simulink model "PIDControls"  (R2024a)
settings: Solver=VariableStepAuto  StartTime=0.0  StopTime=220  RelTol=1e-3
model workspace (MATLAB code in the model file):
  | load('DesiredPitch.mat', '-ascii');
  | load('MeasuredPitch.mat', '-ascii');
  | load('MotorPitchSpeed.mat', '-ascii');
libraries: simulink x6, slpidlib x3, mcbhdlpositiondecoderlib x3
settings Model: Creator=brend  LastModifiedBy=brend

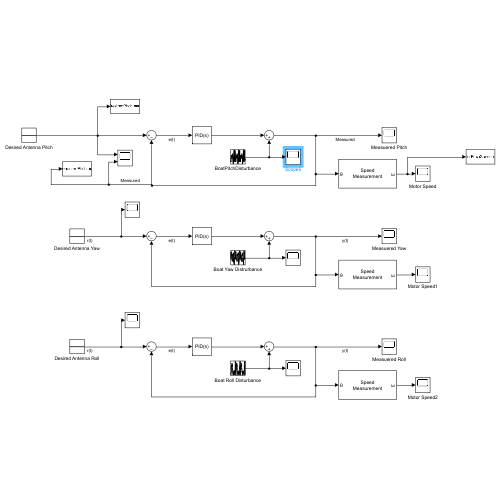
[thumbnail: Simulink's stored preview of the top-level diagram]
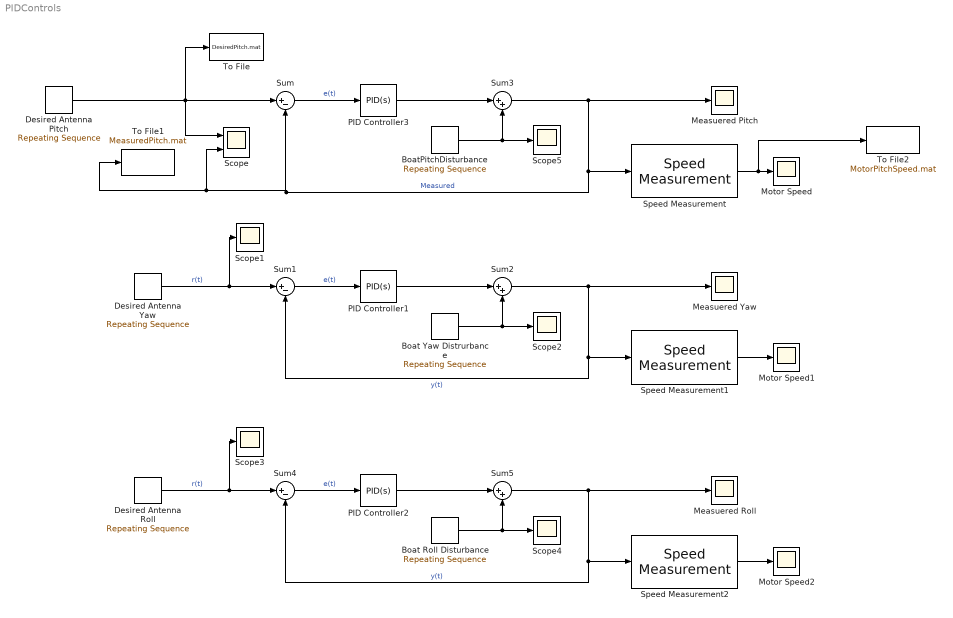
== system PIDControls ==
  Boat Roll Disturbance : simulink/Sources/Repeating Sequence  rep_seq_t=[0:219]  rep_seq_y=|
      | [-14.82
      | -14.76
      | -14.44
      | -13.69
      | -13.53
      | -13.69
      | -13.93
      | -12.12
      | -11.59
      | -10.70
      | -9.70
      | -8.71
      | -8.04
      | -7.18
      | -7.72
      | -7.28
      | -6.48
      | -6.82
      | -5.69
      | -4.25
      | -3.67
      | -2.77
      | 4.98
      | 1.24
      | 2.72
      | 3.04
      | 5.30
      | 5.55
      | 6.34
      | 5.33
      | 4.86
      | 4.27
      | 3.96
      | 3.72
      | 3.36
      | 3.85
      | 3.34
      | 3.19
      | 3.12
      | 4.38
      | 5.56
      | 6.85
      | 8.98
      | 8.41
      | 10.12
      | 10.66
      | 10.62
      | 10.05
      | 10.68
      | 10.99
      | 9.31
      | 9.86
      | 9.73
      |  9.94
      |  9.40
      |  8.03
      |  8.72
      |  8.40
      |  8.06
      |  8.71
      |  8.34
      |  8.92
      |  7.35
      | 7.33
      | 7.25
      | 6.62
      | 5.37
      | 2.19
      | 1.43
      | -3.62
      | -4.20
      | -4.94
      | -5.09
      | -4.96
      | -4.24
      | -4.35
      | -4.67
      | -4.65
      | -4.90
      | -4.35
      | -5.32
      | -6.85
      | -7.31
      | -8.65
      | -9.51
      | -9.25
      | -9.49
      | -8.63
      | -7.78
      | -7.82
      | -6.51
      | -6.54
      | -6.65
      | -6.65
      | -6.33
      | -7.93
      | -8.33
      | -10.03
      | -10.99
      | -11.75
      | -12.80
      | -12.82
      | -13.35
      | -13.70
      | -14.00
      | -14.19
      | -14.98
      | -15.90
      | -15.33
      | -15.71
      | -15.71
      | -14.54
      | -13.07
      |  -13.51
      |  -12.82
      |  -12.40
      |  -11.25
      |  -11.17
      |  -11.99
      |  -11.62
      |  -11.31
      |  -11.53
      |  -14.76
      |  -9.06
      |  -8.28
      | -7.97
      |  -7.84
      |  -8.19
      |  -8.18
      |  -9.32
      |  -10.31
      |  -11.65
      |  -12.48
      |  -13.99
      |  -13.11
      |  -14.27
      |  -13.54
      |  -14.41
      |  -13.38
      |  -9.72
      |  -7.96
      |  -6.05
      |  -5.00
      |  -5.70
      |  -5.78
      |  -5.59
      |  -5.76
      |  -5.11
      |  -5.50
      |  -5.89
      |  -5.28
      |  -5.76
      |  -5.48
      |  -5.73
      |  -6.97
      |  -6.88
      |  -7.37
      | -8.31
      | -9.30
      | -10.64
      | -11.10
      | -12.63
      | -12.95
      | -13.27
      | -13.87
      | -13.60
      | -13.99
      | -17.11
      | -13.40
      | -11.64
      | -10.60
      |  -10.77
      |  -10.26
      |  -11.02
      |  -11.54
      |  -11.51
      |  -11.68
      |  -11.79
      |  -10.58
      |  -10.79
      |  -10.15
      |  -9.59
      |  -8.36
      |  -7.25
      |  -6.32
      |  -5.45
      |  -4.09
      |  -4.25
      |  -3.73
      |  -3.28
      |  -3.67
      |  -2.62
      |  -2.80
      | -2.70
      | -2.38
      |  1.01
      |  2.23
      |  2.11
      |  4.37
      |  6.51
      |  7.00
      |  7.75
      |  8.28
      |  8.00
      |  9.87
      |  10.54
      |  10.20
      |  11.15
      |  13.65
      |  13.74
      |  14.26
      |  14.88
      |  14.77
      |  13.66
      |  12.22
      |  12.93
      |  11.12
      |  12.36
      |  12.25
      |  14.61]
  Boat Yaw Distrurbance : simulink/Sources/Repeating Sequence  rep_seq_t=[0:219]  rep_seq_y=|
      | [-5.64 
      | -4.89 
      | -3.70 
      | -2.04 
      | 0.07  
      | 2.54  
      | 5.24  
      | 7.96  
      | 10.51 
      | 12.70 
      | 14.35 
      | 15.35 
      | 15.66 
      | 15.27 
      | 14.23 
      | 12.65 
      | 10.67 
      | 8.48  
      | 6.28  
      | 4.24  
      | 2.51  
      | 1.16  
      | 0.21  
      | -0.38 
      | -0.68 
      | -0.81 
      | -0.86 
      | -0.92 
      | -1.06 
      | -1.29 
      | -1.62 
      | -1.99 
      | -2.37 
      | -2.70 
      | -2.94 
      | -3.08 
      | -3.14 
      | -3.15 
      | -3.15 
      | -3.22 
      | -3.40 
      | -3.72 
      | -4.21 
      | -4.84 
      | -5.58 
      | -6.37 
      | -7.15 
      | -7.86 
      | -8.47 
      | -8.95 
      | -9.32 
      | -9.59 
      | -9.81 
      | -10.01
      | -10.24
      | -10.51
      | -10.83
      | -11.15
      | -11.43
      | -11.58
      | -11.53
      | -11.20
      | -10.50
      | -9.40 
      | -7.90 
      | -6.02 
      | -3.83 
      | -1.47 
      | 0.92  
      | 3.18  
      | 5.15  
      | 6.72  
      | 7.81  
      | 8.39  
      | 8.48  
      | 8.16  
      | 7.53  
      | 6.73  
      | 5.90  
      | 5.18  
      | 4.67  
      | 4.44  
      | 4.50  
      | 4.81  
      |  5.31 
      |  5.88 
      |  6.43 
      | 6.86  
      | 7.10  
      | 7.14  
      | 7.01  
      | 6.76  
      | 6.49  
      | 6.29  
      | 6.25  
      | 6.43  
      | 6.85  
      |  7.45 
      |  8.17 
      |  8.87 
      |  9.43 
      |  9.75 
      |  9.75 
      |  9.40 
      |  8.75 
      |  7.89 
      |  6.98 
      |  6.21 
      |  5.73 
      |  5.71 
      |  6.20 
      |  7.21 
      |  8.61 
      |  10.22
      |  11.78
      |  13.04
      |  13.74
      |  13.69
      |  12.77
      |  10.92
      |  8.22 
      |  4.82 
      |  1.01 
      |  -2.85
      | -6.39 
      | -9.30 
      | -11.37
      | -12.50
      | -12.70
      | -12.07
      | -10.76
      | -9.00 
      | -7.06 
      | -5.22 
      | -3.72 
      | -2.76 
      | -2.46 
      | -2.85 
      | -3.92 
      | -5.58 
      | -7.68 
      | -10.06
      | -12.54
      | -14.95
      | -17.15
      | -19.00
      | -20.43
      | -21.38
      | -21.81
      | -21.71
      | -21.11
      | -20.05
      | -18.59
      | -16.85
      | -14.95
      | -13.06
      | -11.30
      | -9.79 
      | -8.61 
      | -7.77 
      | -7.20 
      | -6.82 
      | -6.46 
      | -5.97 
      | -5.21 
      | -4.05 
      | -2.43 
      | -0.34 
      |  2.13 
      |  4.88 
      |  7.73 
      |  10.50
      |  13.02
      |  15.18
      |  16.90
      |  18.15
      |  18.94
      |  19.33
      |  19.36
      |  19.09
      |  18.59
      |  17.90
      | 17.06 
      | 16.10 
      | 15.04 
      |  13.89
      |  12.67
      |  11.41
      |  10.12
      |  8.84 
      |  7.57 
      |  6.33 
      |  5.10 
      | 3.89  
      | 2.67  
      | 1.43  
      | 0.16  
      | -1.12 
      | -2.38 
      | -3.56 
      | -4.59 
      | -5.40 
      | -5.94 
      | -6.16 
      | -6.07 
      | -5.70 
      | -5.14 
      | -4.49 
      | -3.85 
      | -3.32 
      | -2.99 
      | -2.89 
      | -2.99 
      | -3.25 
      | -3.56 
      | -3.82 
      | -3.94 
      | -3.85 
      | -3.52 
      | -2.98 ]
  BoatPitchDisturbance : simulink/Sources/Repeating Sequence  rep_seq_t=[0:219]  rep_seq_y=|
      | [-6.01
      | -7.17
      | -8.05
      | -8.55
      | -8.58
      | -8.11
      | -7.17
      | -5.83
      | -4.20
      | -2.44
      | -0.69
      | 0.91 
      | 2.25 
      | 3.27 
      | 3.96 
      | 4.35 
      | 4.47 
      | 4.38 
      | 4.14 
      | 3.79 
      | 3.37 
      | 2.90 
      | 2.40 
      | 1.90 
      | 1.42 
      | 1.00 
      | 0.69 
      | 0.54 
      | 0.60 
      | 0.90 
      | 1.41 
      | 2.12 
      | 2.93 
      | 3.75 
      | 4.46 
      | 4.96 
      | 5.15 
      | 4.99 
      | 4.48 
      | 3.65 
      | 2.60 
      | 1.44 
      | 0.30 
      | -0.72
      | -1.51
      | -2.04
      | -2.28
      | -2.27
      | -2.08
      | -1.75
      | -1.37
      | -0.99
      | -0.65
      | -0.34
      | -0.07
      | 0.18 
      | 0.44 
      | 0.71 
      | 1.00 
      | 1.30 
      | 1.57 
      | 1.81 
      | 2.00 
      | 2.13 
      | 2.24 
      | 2.36 
      | 2.55 
      | 2.86 
      | 3.33 
      | 3.98 
      | 4.77 
      | 5.66 
      | 6.55 
      | 7.32 
      | 7.85 
      | 8.06 
      | 7.88 
      | 7.30 
      | 6.35 
      | 5.12 
      | 3.74 
      | 2.38 
      | 1.18 
      | 0.28 
      | -0.23
      | -0.34
      | -0.05
      | 0.53 
      | 1.29 
      | 2.08 
      | 2.77 
      | 3.23 
      | 3.36 
      | 3.12 
      | 2.49 
      | 1.50 
      | 0.20 
      | -1.33
      | -2.99
      | -4.69
      | -6.35
      | -7.88
      | -9.21
      | -10.32
      | -11.14
      | -11.75
      | -11.93
      | -11.97
      | -11.84
      | -11.45
      | -10.95
      | -10.43
      | -9.91
      | -9.38
      | -8.88
      | -8.36
      | -7.80
      | -7.13
      | -6.30
      | -5.29
      | -4.08
      | -2.73
      | -1.33
      | -0.00
      | 1.10 
      | 1.83 
      | 2.06 
      | 1.74 
      | 0.86 
      | -0.50
      | -2.18
      | -3.97
      | -5.62
      | -6.91
      | -7.63
      | -7.66
      | -6.92
      | -5.45
      | -3.34
      | -0.76
      | 2.08 
      | 4.94 
      | 7.61 
      | 9.95 
      | 11.85
      | 13.27
      | 14.22
      | 14.73
      | 14.83
      | 14.56
      | 13.93
      | 12.96
      | 11.65
      | 10.02
      | 8.09 
      | 5.93 
      | 3.63 
      | 1.33 
      | -0.81
      | -2.63
      | -4.03
      | -4.90
      | -5.23
      | -5.06
      | -4.51
      | -3.72
      | -2.89
      | -2.20
      | -1.82
      | -1.84
      | -2.32
      | -3.20
      | -4.36
      | -5.64
      | -6.84
      | -7.74
      | -8.16
      | -7.98
      | -7.12
      | -5.59
      | -3.45
      | -0.84
      | 2.04 
      | 4.96 
      | 7.69 
      | 10.02
      | 11.80
      | 12.96
      | 13.46
      | 13.33
      | 12.63
      | 11.49
      | 10.03
      | 8.41 
      | 6.80 
      | 5.31 
      | 4.05 
      | 3.07 
      | 2.35 
      | 1.86 
      | 1.50 
      | 1.18 
      | 0.81 
      | 0.32 
      | -0.31
      | -1.06
      | -1.90
      | -2.72
      | -3.42
      | -3.92
      | -4.16
      | -4.10
      | -3.80
      | -3.32
      | -2.80
      | -2.38
      | -2.20
      | -2.35
      | -2.88
      | -3.76]
  "Desired Antenna Pitch " : simulink/Sources/Repeating Sequence  rep_seq_t=[0:219]  rep_seq_y=linspace(30, 30, 220);
  Desired Antenna Roll : simulink/Sources/Repeating Sequence  rep_seq_t=[0:219]  rep_seq_y=linspace(30, 30, 220);
  Desired Antenna Yaw : simulink/Sources/Repeating Sequence  rep_seq_t=[0:219]  rep_seq_y=linspace(30, 30, 220);
  Measuered Pitch : Scope
  Measuered Roll : Scope
  Measuered Yaw : Scope
  Motor Speed : Scope
  Motor Speed1 : Scope
  Motor Speed2 : Scope
  PID Controller1 : slpidlib/PID Controller  Controller=PID  Form=Parallel  TimeDomain=Continuous-time  UseExternalTs=off  SampleTime=-1  IntegratorMethod=Forward Euler  FilterMethod=Forward Euler  ControllerParametersSource=internal  P=1  I=10  UseKiTs=off  D=0  UseExternalDerivativeSource=off  N=100  UseFilter=on  TunerSelectOption=Transfer Function Based (PID Tuner App)  InitialConditionSource=internal  InitialConditionForIntegrator=0  InitialConditionForFilter=0  DifferentiatorICPrevScaledInput=0  ExternalReset=none  TrackingMode=off  Kt=1  LimitOutput=off  SatLimitsSource=internal  UpperSaturationLimit=inf  LowerSaturationLimit=-inf  LinearizeAsGain=on  AntiWindupMode=none  Kb=1  LimitIntegrator=off  UpperIntegratorSaturationLimit=inf  LowerIntegratorSaturationLimit=-inf  POutMin=[]  POutMax=[]  IOutMin=[]  IOutMax=[]  DOutMin=[]  DOutMax=[]  NOutMin=[]  NOutMax=[]  SumOutMin=[]  SumOutMax=[]  SaturationOutMin=[]  SaturationOutMax=[]  PParamMin=[]  PParamMax=[]  IParamMin=[]  IParamMax=[]  DParamMin=[]  DParamMax=[]  NParamMin=[]  NParamMax=[]  KbParamMin=[]  KbParamMax=[]  KtParamMin=[]  KtParamMax=[]  KbOutMin=[]  KbOutMax=[]  KtOutMin=[]  KtOutMax=[]  IntegratorOutMin=[]  IntegratorOutMax=[]  FilterOutMin=[]  FilterOutMax=[]  SumI1OutMin=[]  SumI1OutMax=[]  SumI2OutMin=[]  SumI2OutMax=[]  SumI3OutMin=[]  SumI3OutMax=[]  SumI4OutMin=[]  SumI4OutMax=[]  SumDOutMin=[]  SumDOutMax=[]  DifferentiatorOutMin=[]  DifferentiatorOutMax=[]  FilterDiffOutCoefMin=[]  FilterDiffOutCoefMax=[]  ReciprocalOutMin=[]  ReciprocalOutMax=[]  SumDenOutMin=[]  SumDenOutMax=[]  SumNumOutMin=[]  SumNumOutMax=[]  DivideOutMin=[]  DivideOutMax=[]  UdiffTsProdOutMin=[]  UdiffTsProdOutMax=[]  NTsProdOutMin=[]  NTsProdOutMax=[]  UintegralTsProdOutMin=[]  UintegralTsProdOutMax=[]  UngainTsProdOutMin=[]  UngainTsProdOutMax=[]  ClampingZeroOutDataTypeStr=Inherit: Inherit via back propagation  ClampingZeroOutMin=[]  ClampingZeroOutMax=[]  FilterDenConstantOutDataTypeStr=Inherit: Inherit via back propagation  FilterDenConstantOutMin=[]  FilterDenConstantOutMax=[]  PCopyOutDataTypeStr=Inherit: Inherit via back propagation  PCopyOutMin=[]  PCopyOutMax=[]  NCopyOutDataTypeStr=Inherit: Inherit via back propagation  NCopyOutMin=[]  NCopyOutMax=[]  IntegratorContinuousStateAttributes=''  IntegratorStateMustResolveToSignalObject=off  IntegratorRTWStateStorageClass=Auto  FilterContinuousStateAttributes=''  FilterStateMustResolveToSignalObject=off  FilterRTWStateStorageClass=Auto  ParallelPVariant=InternalParameters  IdealPVariant=Disabled  IVariant=InternalParameters  DVariant=InternalParameters  IntegratorVariant=Continuous  SatVariant=Disabled  AWVariant=Passthrough  PCopyVariant=Disabled  TRVariant=Disabled  FdbkBlocksVariant=Forward  IdealPFdbkVariant=Disabled  SatFdbkVariant=Disabled  DerivativeFilterVariant=ContFilter  NVariant=InternalParameters  NCopyVariant=Disabled  FilterICVariant=InternalICsFilter  IntegratorICVariant=InternalICs  ExternalResetVariant=Disabled  TRSumVariant=Passthrough  SumFdbkVariant=Disabled  SumVariant=Sum_PID  TsampFilterVariant=InternalTs  TsampNgainVariant=Passthrough  TsampIntegralVariant=Disabled_SignalSpec  ExternalSaturationOutDataTypeStr=Inherit: Same as second input  DerivativeSourceVariant=ErrorSignal
  PID Controller2 : slpidlib/PID Controller  Controller=PID  Form=Parallel  TimeDomain=Continuous-time  UseExternalTs=off  SampleTime=-1  IntegratorMethod=Forward Euler  FilterMethod=Forward Euler  ControllerParametersSource=internal  P=1  I=10  UseKiTs=off  D=0  UseExternalDerivativeSource=off  N=100  UseFilter=on  TunerSelectOption=Transfer Function Based (PID Tuner App)  InitialConditionSource=internal  InitialConditionForIntegrator=0  InitialConditionForFilter=0  DifferentiatorICPrevScaledInput=0  ExternalReset=none  TrackingMode=off  Kt=1  LimitOutput=off  SatLimitsSource=internal  UpperSaturationLimit=inf  LowerSaturationLimit=-inf  LinearizeAsGain=on  AntiWindupMode=none  Kb=1  LimitIntegrator=off  UpperIntegratorSaturationLimit=inf  LowerIntegratorSaturationLimit=-inf  POutMin=[]  POutMax=[]  IOutMin=[]  IOutMax=[]  DOutMin=[]  DOutMax=[]  NOutMin=[]  NOutMax=[]  SumOutMin=[]  SumOutMax=[]  SaturationOutMin=[]  SaturationOutMax=[]  PParamMin=[]  PParamMax=[]  IParamMin=[]  IParamMax=[]  DParamMin=[]  DParamMax=[]  NParamMin=[]  NParamMax=[]  KbParamMin=[]  KbParamMax=[]  KtParamMin=[]  KtParamMax=[]  KbOutMin=[]  KbOutMax=[]  KtOutMin=[]  KtOutMax=[]  IntegratorOutMin=[]  IntegratorOutMax=[]  FilterOutMin=[]  FilterOutMax=[]  SumI1OutMin=[]  SumI1OutMax=[]  SumI2OutMin=[]  SumI2OutMax=[]  SumI3OutMin=[]  SumI3OutMax=[]  SumI4OutMin=[]  SumI4OutMax=[]  SumDOutMin=[]  SumDOutMax=[]  DifferentiatorOutMin=[]  DifferentiatorOutMax=[]  FilterDiffOutCoefMin=[]  FilterDiffOutCoefMax=[]  ReciprocalOutMin=[]  ReciprocalOutMax=[]  SumDenOutMin=[]  SumDenOutMax=[]  SumNumOutMin=[]  SumNumOutMax=[]  DivideOutMin=[]  DivideOutMax=[]  UdiffTsProdOutMin=[]  UdiffTsProdOutMax=[]  NTsProdOutMin=[]  NTsProdOutMax=[]  UintegralTsProdOutMin=[]  UintegralTsProdOutMax=[]  UngainTsProdOutMin=[]  UngainTsProdOutMax=[]  ClampingZeroOutDataTypeStr=Inherit: Inherit via back propagation  ClampingZeroOutMin=[]  ClampingZeroOutMax=[]  FilterDenConstantOutDataTypeStr=Inherit: Inherit via back propagation  FilterDenConstantOutMin=[]  FilterDenConstantOutMax=[]  PCopyOutDataTypeStr=Inherit: Inherit via back propagation  PCopyOutMin=[]  PCopyOutMax=[]  NCopyOutDataTypeStr=Inherit: Inherit via back propagation  NCopyOutMin=[]  NCopyOutMax=[]  IntegratorContinuousStateAttributes=''  IntegratorStateMustResolveToSignalObject=off  IntegratorRTWStateStorageClass=Auto  FilterContinuousStateAttributes=''  FilterStateMustResolveToSignalObject=off  FilterRTWStateStorageClass=Auto  ParallelPVariant=InternalParameters  IdealPVariant=Disabled  IVariant=InternalParameters  DVariant=InternalParameters  IntegratorVariant=Continuous  SatVariant=Disabled  AWVariant=Passthrough  PCopyVariant=Disabled  TRVariant=Disabled  FdbkBlocksVariant=Forward  IdealPFdbkVariant=Disabled  SatFdbkVariant=Disabled  DerivativeFilterVariant=ContFilter  NVariant=InternalParameters  NCopyVariant=Disabled  FilterICVariant=InternalICsFilter  IntegratorICVariant=InternalICs  ExternalResetVariant=Disabled  TRSumVariant=Passthrough  SumFdbkVariant=Disabled  SumVariant=Sum_PID  TsampFilterVariant=InternalTs  TsampNgainVariant=Passthrough  TsampIntegralVariant=Disabled_SignalSpec  ExternalSaturationOutDataTypeStr=Inherit: Same as second input  DerivativeSourceVariant=ErrorSignal
  PID Controller3 : slpidlib/PID Controller  Controller=PID  Form=Parallel  TimeDomain=Continuous-time  UseExternalTs=off  SampleTime=-1  IntegratorMethod=Forward Euler  FilterMethod=Forward Euler  ControllerParametersSource=internal  P=1  I=10  UseKiTs=off  D=0  UseExternalDerivativeSource=off  N=100  UseFilter=on  TunerSelectOption=Transfer Function Based (PID Tuner App)  InitialConditionSource=internal  InitialConditionForIntegrator=0  InitialConditionForFilter=0  DifferentiatorICPrevScaledInput=0  ExternalReset=none  TrackingMode=off  Kt=1  LimitOutput=off  SatLimitsSource=internal  UpperSaturationLimit=inf  LowerSaturationLimit=-inf  LinearizeAsGain=on  AntiWindupMode=none  Kb=1  LimitIntegrator=off  UpperIntegratorSaturationLimit=inf  LowerIntegratorSaturationLimit=-inf  POutMin=[]  POutMax=[]  IOutMin=[]  IOutMax=[]  DOutMin=[]  DOutMax=[]  NOutMin=[]  NOutMax=[]  SumOutMin=[]  SumOutMax=[]  SaturationOutMin=[]  SaturationOutMax=[]  PParamMin=[]  PParamMax=[]  IParamMin=[]  IParamMax=[]  DParamMin=[]  DParamMax=[]  NParamMin=[]  NParamMax=[]  KbParamMin=[]  KbParamMax=[]  KtParamMin=[]  KtParamMax=[]  KbOutMin=[]  KbOutMax=[]  KtOutMin=[]  KtOutMax=[]  IntegratorOutMin=[]  IntegratorOutMax=[]  FilterOutMin=[]  FilterOutMax=[]  SumI1OutMin=[]  SumI1OutMax=[]  SumI2OutMin=[]  SumI2OutMax=[]  SumI3OutMin=[]  SumI3OutMax=[]  SumI4OutMin=[]  SumI4OutMax=[]  SumDOutMin=[]  SumDOutMax=[]  DifferentiatorOutMin=[]  DifferentiatorOutMax=[]  FilterDiffOutCoefMin=[]  FilterDiffOutCoefMax=[]  ReciprocalOutMin=[]  ReciprocalOutMax=[]  SumDenOutMin=[]  SumDenOutMax=[]  SumNumOutMin=[]  SumNumOutMax=[]  DivideOutMin=[]  DivideOutMax=[]  UdiffTsProdOutMin=[]  UdiffTsProdOutMax=[]  NTsProdOutMin=[]  NTsProdOutMax=[]  UintegralTsProdOutMin=[]  UintegralTsProdOutMax=[]  UngainTsProdOutMin=[]  UngainTsProdOutMax=[]  ClampingZeroOutDataTypeStr=Inherit: Inherit via back propagation  ClampingZeroOutMin=[]  ClampingZeroOutMax=[]  FilterDenConstantOutDataTypeStr=Inherit: Inherit via back propagation  FilterDenConstantOutMin=[]  FilterDenConstantOutMax=[]  PCopyOutDataTypeStr=Inherit: Inherit via back propagation  PCopyOutMin=[]  PCopyOutMax=[]  NCopyOutDataTypeStr=Inherit: Inherit via back propagation  NCopyOutMin=[]  NCopyOutMax=[]  IntegratorContinuousStateAttributes=''  IntegratorStateMustResolveToSignalObject=off  IntegratorRTWStateStorageClass=Auto  FilterContinuousStateAttributes=''  FilterStateMustResolveToSignalObject=off  FilterRTWStateStorageClass=Auto  ParallelPVariant=InternalParameters  IdealPVariant=Disabled  IVariant=InternalParameters  DVariant=InternalParameters  IntegratorVariant=Continuous  SatVariant=Disabled  AWVariant=Passthrough  PCopyVariant=Disabled  TRVariant=Disabled  FdbkBlocksVariant=Forward  IdealPFdbkVariant=Disabled  SatFdbkVariant=Disabled  DerivativeFilterVariant=ContFilter  NVariant=InternalParameters  NCopyVariant=Disabled  FilterICVariant=InternalICsFilter  IntegratorICVariant=InternalICs  ExternalResetVariant=Disabled  TRSumVariant=Passthrough  SumFdbkVariant=Disabled  SumVariant=Sum_PID  TsampFilterVariant=InternalTs  TsampNgainVariant=Passthrough  TsampIntegralVariant=Disabled_SignalSpec  ExternalSaturationOutDataTypeStr=Inherit: Same as second input  DerivativeSourceVariant=ErrorSignal
  Scope : Scope  NumInputPorts=2
  Scope{1..5} (5 alike) : Scope
  Speed Measurement : mcbhdlpositiondecoderlib/Speed Measurement  PositionUnit=Radians  PositionScalingDatatype=uint32  SpeedCalculationMode=Maximum application speed  SampleTimeAsync=100e-6  MaximumApplicationSpeed=1000  SpeedResolution=5e-6  DelayLength=299  MaximumMeasurableSpeed=1000  MeasurableSpeedResolution=4.6566e-07  SpeedUnit=RPM  PerUnitSpeed=1000  SpeedDataType=single
      settings: LibrarySourceBlock=mcbhdllib/Sensor Decoders/Speed Measurement
  Speed Measurement1 : mcbhdlpositiondecoderlib/Speed Measurement  PositionUnit=Radians  PositionScalingDatatype=uint32  SpeedCalculationMode=Maximum application speed  SampleTimeAsync=100e-6  MaximumApplicationSpeed=1000  SpeedResolution=5e-6  DelayLength=299  MaximumMeasurableSpeed=1000  MeasurableSpeedResolution=4.6566e-07  SpeedUnit=RPM  PerUnitSpeed=1000  SpeedDataType=single
      settings: LibrarySourceBlock=mcbhdllib/Sensor Decoders/Speed Measurement
  Speed Measurement2 : mcbhdlpositiondecoderlib/Speed Measurement  PositionUnit=Radians  PositionScalingDatatype=uint32  SpeedCalculationMode=Maximum application speed  SampleTimeAsync=100e-6  MaximumApplicationSpeed=1000  SpeedResolution=5e-6  DelayLength=299  MaximumMeasurableSpeed=1000  MeasurableSpeedResolution=4.6566e-07  SpeedUnit=RPM  PerUnitSpeed=1000  SpeedDataType=single
      settings: LibrarySourceBlock=mcbhdllib/Sensor Decoders/Speed Measurement
  Sum : Sum  Inputs=|+-
  Sum1 : Sum  Inputs=|+-
  Sum2 : Sum  Inputs=|++
  Sum3 : Sum  Inputs=|++
  Sum4 : Sum  Inputs=|+-
  Sum5 : Sum  Inputs=|++
  To File : ToFile  Filename=DesiredPitch.mat  MatrixName=DesiredPitch  SaveFormat=Timeseries
  To File1 : ToFile  Filename=MeasuredPitch.mat  MatrixName=MeasuredPitch  SaveFormat=Timeseries
  To File2 : ToFile  Filename=MotorPitchSpeed.mat  MatrixName=MotorPitchSpeed  SaveFormat=Timeseries
  wires:
  Sum/1 -> PID Controller3/1  "e(t)"
  Sum3/1 -> Measuered Pitch/1, To File1/1, Scope/2, Sum/2, Speed Measurement/1  "Measured"
  PID Controller3/1 -> Sum3/1
  BoatPitchDisturbance/1 -> Scope5/1, Sum3/2
  Speed Measurement/1 -> To File2/1, Motor Speed/1
  Speed Measurement1/1 -> Motor Speed1/1
  Sum1/1 -> PID Controller1/1  "e(t)"
  PID Controller1/1 -> Sum2/1
  Boat Yaw Distrurbance/1 -> Scope2/1, Sum2/2
  Desired Antenna Yaw/1 -> Scope1/1, Sum1/1  "r(t)"
  Sum2/1 -> Measuered Yaw/1, Sum1/2, Speed Measurement1/1  "y(t)"
  Speed Measurement2/1 -> Motor Speed2/1
  Sum4/1 -> PID Controller2/1  "e(t)"
  PID Controller2/1 -> Sum5/1
  Boat Roll Disturbance/1 -> Scope4/1, Sum5/2
  Desired Antenna Roll/1 -> Sum4/1, Scope3/1  "r(t)"
  Sum5/1 -> Measuered Roll/1, Sum4/2, Speed Measurement2/1  "y(t)"
  "Desired Antenna Pitch "/1 -> To File/1, Scope/1, Sum/1
